simulink model "firdecimation_ref3"  (Simulink 4.00)
settings: Solver=FixedStepDiscrete  SolverMode=MultiTasking  StartTime=0.0  StopTime=30  RelTol=1e-3
PostLoadFcn:
  | set_param(gcs,'SimulationCommand','Update')
libraries: dspmlti3 x1, dspsrcs3 x1
settings Model: RequirementInfo=9  LastModifiedBy=dfass  LimitDataPoints=off  ExtModeTrigMode=oneshot  ExtModeArmWhenConnect=off  BlockReductionOpt=off

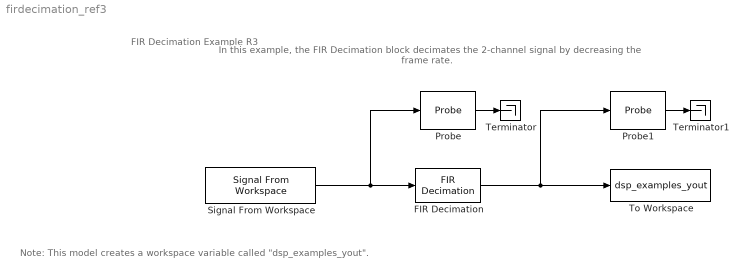
== system firdecimation_ref3 ==
  note: FIR Decimation Example R3
  note: In this example, the FIR Decimation block decimates the
      | 2-channel signal by decreasing the frame rate.
  note: Note: This model creates a workspace variable called "dsp_examples_yout".
  FIR Decimation : dspmlti3/FIR Decimation  h=fir1(3,0.25)  D=2  framing=Maintain input frame size
  Probe : Probe  ProbeWidth=off  ProbeSampleTime=on  ProbeComplexSignal=off  ProbeSignalDimensions=off
  Probe1 : Probe  ProbeWidth=off  ProbeSampleTime=on  ProbeComplexSignal=off  ProbeSignalDimensions=off
  Signal From Workspace : dspsrcs3/Signal From Workspace  X=[(1:100)' (-1:-1:-100)']  Ts=0.25  nsamps=4  OutputAfterFinalValue=Setting To Zero
  Terminator : Terminator
  Terminator1 : Terminator
  To Workspace : ToWorkspace  VariableName=dsp_examples_yout  SampleTime=-1  SaveFormat=Array
  wires:
  FIR Decimation/1 -> To Workspace/1, Probe1/1
  Signal From Workspace/1 -> Probe/1, FIR Decimation/1
  Probe/1 -> Terminator/1
  Probe1/1 -> Terminator1/1
